simulink model "simulink_sim"  (R2017a)
settings: Solver=VariableStepAuto  StartTime=0.0  StopTime=10.0  RelTol=1e-3
libraries: dsparch4 x1, dspvision x1
settings Model: Creator=Asaf  LastModifiedBy=Asaf

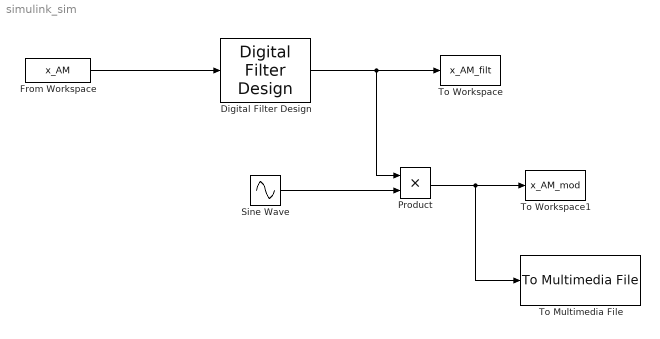
== system simulink_sim ==
  Digital Filter Design : dsparch4/Digital Filter Design  mwdsp_browser_bugfix_var=off
  From Workspace : FromWorkspace  VariableName=x_AM  SampleTime=1/80000
  Product : Product
  Sine Wave : Sin  Amplitude=2  Frequency=2*pi*30000  Phase=pi/2  SampleTime=1/80000
  To Multimedia File : dspvision/To Multimedia File  outputFilename=output.wav  streamSelection=Audio only  videoCompressor=None (uncompressed)  audioCompressor=None (uncompressed)  imagePorts=Separate color signals  fileType=WAV  audioDatatype=16-bit integer  fourcc=RGB  videoQuality=75  mj2000CompFactor=10
      settings: SourceProductName=Computer Vision System Toolbox  SourceProductBaseCode=VP
  To Workspace : ToWorkspace  VariableName=x_AM_filt  SaveFormat=Timeseries  SampleTime=-1
  To Workspace1 : ToWorkspace  VariableName=x_AM_mod  SaveFormat=Timeseries  SampleTime=-1
  wires:
  From Workspace/1 -> Digital Filter Design/1
  Digital Filter Design/1 -> Product/1, To Workspace/1
  Sine Wave/1 -> Product/2
  Product/1 -> To Multimedia File/1, To Workspace1/1
